simulink model "Loops5"  (Simulink 6.0)
settings: Solver=ode45  StartTime=0.0  StopTime=10.0  RelTol=1e-3
settings Model: Creator=scaife  LastModifiedBy=scaife  ExtModeAutoUpdateStatusClock=off
settings DataIOCC: SignalLoggingName=sigsOut
settings DebuggingCC: SolverPrmCheckMsg=none
settings HardwareCC: TargetUnknown=on
settings GRTTargetCC: ModelReferenceCompliant=off  MatFileLogging=off

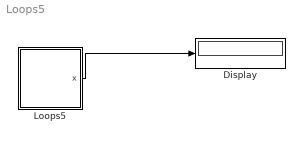
== system Loops5 ==
  Display : Display
  Loops5 : Stateflow chart
  wires:
  Loops5/1(x) -> Display/1

== stateflow chart Loops5 ==
  state A
  state B
  A -> (junction 5) : {x=0;}
  (junction 6) -> B
  (default) -> A : {y=0;}
  (junction 7) -> B
  (junction 5) -> (junction 6) : [y==0]
  (junction 5) -> (junction 7) : [y==1]
  (junction 7) -> (junction 7) : [x<5]
      | {x++;}
  (junction 6) -> (junction 5) : [x<10]
      | {x++;}
  B -> A : {y=(y+1)%%2;}
  data: x output int32; y local int32
